simulink model "Wischer_Sensorbox"  (R2017b)
settings: Solver=FixedStepAuto  StartTime=0.0  StopTime=10.0  RelTol=1e-3
PreLoadFcn:
  | waijung.modelPreload; % Required for working with Waijung Blockset. Do not remove.
undefined symbols (not defined in the file): Blocking, HSEOSC, Link, LQFP100, Non, Raw, ST, STM32F407VG
libraries: simulink x14, hdlsllib x12, stm32f4_canbus_lib x3, stm32f4_io_lib x2, stm32f4_adc_lib x1, stm32f4_device_config_lib x1
CloseFcn:
  | waijung.modelClose; % Required for working with Waijung Blockset. Do not remove.
settings Model: Creator=Alexander  LastModifiedBy=labuser
settings OptimizationCC: DefaultParameterBehavior=Inlined
settings DebuggingCC: ParameterTunabilityLossMsg=error
settings HardwareCC: ProdBitPerPointer=32  ProdBitPerSizeT=32  ProdBitPerPtrDiffT=32  ProdLargestAtomicFloat=None  ProdIntDivRoundTo=Undefined  ProdWordSize=32  ProdHWDeviceType=ARM Compatible->Cortex - M4  TargetEndianess=LittleEndian  TargetHWDeviceType=ARM Compatible->Cortex - M4
settings SFSimCC: MATLABDynamicMemAlloc=off
settings RTWCC: SystemTargetFile=stm32f4.tlc  GenerateMakefile=off  TemplateMakefile=ert_default_tmf  Description=STM32F4 Target  GenerateReport=on  IncludeHyperlinkInReport=on  LaunchReport=on  GenerateTraceInfo=on  GenerateTraceReport=on  GenerateTraceReportSl=on  GenerateTraceReportSf=on  GenerateTraceReportEml=on
settings CodeAppCC: ForceParamTrailComments=on  IgnoreCustomStorageClasses=off  OperatorAnnotations=on  SimulinkDataObjDesc=on  SFDataObjDesc=on  MATLABFcnDesc=on  InsertBlockDesc=on  StateflowObjectComments=on  MATLABSourceComments=on
settings STFCustomTargetCC: TargetLangStandard=C99 (ISO)  ModelReferenceCompliant=off  CombineOutputUpdateFcns=on  ERTCustomFileBanners=on  SupportContinuousTime=off  SupportNonInlinedSFcns=off  RemoveResetFunc=on  MATLABClassNameForMDSCustomization=Simulink.SoftwareTarget.ERTCustomization  GRTInterface=off  SystemTargetFile=stm32f4.tlc
settings ERTTargetCC: TargetLangStandard=C99 (ISO)  MultiwordLength=2048  ModelReferenceCompliant=off  ParMdlRefBuildCompliant=off  CompOptLevelCompliant=off  ConcurrentExecutionCompliant=off  ModelStepFunctionPrototypeControlCompliant=off  CPPClassGenCompliant=off  UseToolchainInfoCompliant=off  InlinedParameterPlacement=NonHierarchical  ERTSrcFileBannerTemplate=stm32f4_code_template.cgt  ERTHdrFileBannerTemplate=stm32f4_code_template.cgt  ERTDataSrcFileTemplate=stm32f4_code_template.cgt  ERTDataHdrFileTemplate=stm32f4_code_template.cgt  ERTCustomFileTemplate=stm32f4_file_process.tlc

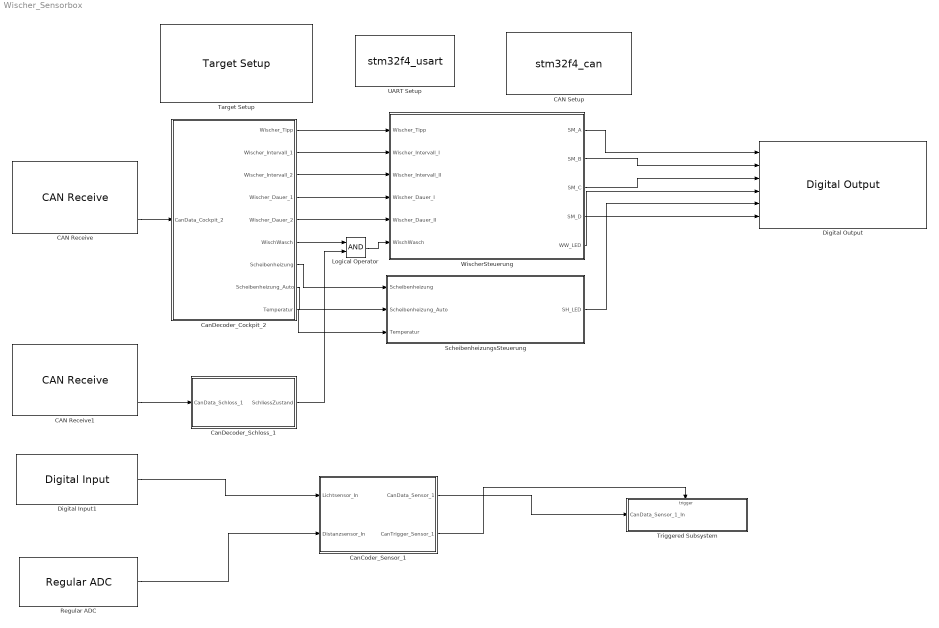
== system Wischer_Sensorbox ==
  CAN Receive : stm32f4_canbus_lib/CAN Receive  conf=Rx  canmodule=1  idtype=Standard  filtertype=Specific  id=17  idmask=0  enableisr=off  usedlc=off  datatype=single  data0type=uint16  data1type=Not used  data2type=Not used  data3type=Not used  data4type=Not used  data5type=Not used  data6type=Not used  data7type=Not used  buffersize=8  sampletime=-1  sampletimestr=-1  blockid=CANReceive  inputarray=[]  inputlabelarray={}  outputarray=[ 5, 7, 5]  outputlabelarray={ 'Msg Pending','ID', 'D0 (uint16)' }  compat=0  confstr="[\"Standard\",\"Specific\",\"17\",\"0\",\"off\",\"uint16\",\"Not used\",\"Not used\",\"Not used\",\"Not used\",\"Not used\",\"Not used\",\"Not used\",\"8\",\"220\",\"0\",\"FFE0\",\"4\"]"
  CAN Receive1 : stm32f4_canbus_lib/CAN Receive  conf=Rx  canmodule=1  idtype=Standard  filtertype=Specific  id=25  idmask=0  enableisr=off  usedlc=off  datatype=single  data0type=uint8  data1type=Not used  data2type=Not used  data3type=Not used  data4type=Not used  data5type=Not used  data6type=Not used  data7type=Not used  buffersize=8  sampletime=-1  sampletimestr=-1  blockid=CANReceive1  inputarray=[]  inputlabelarray={}  outputarray=[ 5, 7, 3]  outputlabelarray={ 'Msg Pending','ID', 'D0 (uint8)' }  compat=0  confstr="[\"Standard\",\"Specific\",\"25\",\"0\",\"off\",\"uint8\",\"Not used\",\"Not used\",\"Not used\",\"Not used\",\"Not used\",\"Not used\",\"Not used\",\"8\",\"320\",\"0\",\"FFE0\",\"4\"]"
  CAN Setup : S-Function  FunctionName=stm32f4_can  Parameters=conf,canmodule,0,inputarray,outputarray,'','',confstr,sampletime,sampletimestr,blockid  SFunctionDeploymentMode=off  EnableBusSupport=off  mask(stm32f4_can){conf=Setup, canmodule=1, advance=off, bitrate_select=125000, sjw=1tq, bs1=14tq, bs2=6tq, timingconf=Prescaler, brp=16, bitrate=125000, tq=3.8095e-07, autoretransmission=Disable, remaptxpin=D1, remaprxpin=D0, sampletime=-1, sampletimestr=-1, blockid=CANSetup, inputarray=[], inputlabelarray={}, outputarray=[], outputlabelarray={}, compat=0, confstr=["125000","16","D","1","D","0","1tq","14tq","6tq","ENABLE"], presc=16, txportstr=D, txpinstr=1, rxportstr=D, rxpinstr=0, lastmodule=1}
      mask prompts: conf "Configuration"; canmodule "CAN Module"; advance "Advance configuration"; bitrate_select "Baud rate (bps)"; sjw "Resync Jump Width (SJW)"; bs1 "Bit segment 1 (BS1) + PROP_SEG"; bs2 "Bit segment 2 (BS2)"; timingconf "Adjust"; brp "Baud rate prescaler (BRP)"; bitrate "Baud rate (bps)"; tq "Time Quantum (Second), tq"; autoretransmission "Auto Re-transmission"; remaptxpin "CAN Tx pin"; remaprxpin "CAN Rx pin"; sampletime "Sample time (sec)"; sampletimestr "Compiled sample time (sec) in string"; inputarray "Input port"; inputlabelarray "Input port label"; outputarray "Output port"; outputlabelarray "Output port label"; compat "Compatibility (Reserved for future use)"; confstr "Configuration String"; presc "Prescale"; txportstr "Tx port string"; txpinstr "Tx pin string"; rxportstr "Rx port string"; rxpinstr "Rx pin string"; lastmodule "Last module selected"
      mask help:
      | This block setups CAN Module.
      |
      | Auto Re-transmission,
      |  - Enable: The CAN hardware will automatically retransmit the message until it has been
      | successfully transmitted according to the CAN standard.
      |  - Disable: A message will be transmitted only once, independently of the transmission result
      | (successful, error or arbitration lost).
      mask init:
      | stm32f4_can_callback('init');
      mask Help: web(fullfile(waijungdocroot,'stm32f4_can_setup.htm'), '-browser')
      mask TypeOptions conf: Setup
      mask TypeOptions canmodule: 1 | 2
      mask Callback canmodule: stm32f4_can_callback('canmodule');
      mask Callback advance: stm32f4_can_callback('advance');
      mask TypeOptions bitrate_select: 125000 | 250000 | 500000 | 1000000
      mask Callback bitrate_select: stm32f4_can_callback('bitrate_select');
      mask TypeOptions sjw: 1tq | 2tq | 3tq | 4tq
      mask TypeOptions bs1: 1tq | 2tq | 3tq | 4tq | 5tq | 6tq | 7tq | 8tq | 9tq | 10tq | 11tq | 12tq | 13tq | 14tq | 15tq | 16tq
      mask Callback bs1: stm32f4_can_callback('timingconf');
      mask TypeOptions bs2: 1tq | 2tq | 3tq | 4tq | 5tq | 6tq | 7tq | 8tq
      mask Callback bs2: stm32f4_can_callback('timingconf');
      mask TypeOptions timingconf: Prescaler | Baudrate
      mask Callback timingconf: stm32f4_can_callback('timingconf');
      mask Callback brp: stm32f4_can_callback('timingconf');
      mask Callback bitrate: stm32f4_can_callback('timingconf');
      mask TypeOptions autoretransmission: Enable | Disable
      mask TypeOptions remaptxpin: Not used | A12 | B9 | D1
      mask Callback remaptxpin: stm32f4_can_callback('remaptxpin');
      mask TypeOptions remaprxpin: Not used | A11 | B8 | D0
      mask Callback remaprxpin: stm32f4_can_callback('remaprxpin');
      mask Callback sampletime: stm32f4_can_callback('sampletime');
      mask Callback sampletimestr: stm32f4_can_callback('sampletimestr');
      mask Callback blockid: stm32f4_can_callback('blockid');
      mask Display: text(0.5, 0.5, 'CAN1_Setup\nSpeed (bps): 125000\nTx/Rx pin: D1/D0','ver','middle','hor','center');
  CanCoder_Sensor_1 : Subsystem
  CanDecoder_Cockpit_2 : Subsystem
  CanDecoder_Schloss_1 : Subsystem
  Digital Input1 : stm32f4_io_lib/Digital Input  port=C  speed=100  porttype=None  porttypestr=NOPULL  use_pin0=off  use_pin1=off  use_pin2=off  use_pin3=off  use_pin4=off  use_pin5=off  use_pin6=on  use_pin7=off  use_pin8=off  use_pin9=off  use_pin10=off  use_pin11=off  use_pin12=off  use_pin13=off  use_pin14=off  use_pin15=off  pinstr=GPIO_Pin_6  usedpinarray="[0  0  0  0  0  0  1  0  0  0  0  0  0  0  0  0]"  bitbandingstr="#define DigitalInput1_C6 Peripheral_BB(GPIOC->IDR, 6)  /* Output pin */"  sampletime=0.01  sampletimestr=-1  blockid=DigitalInput1  enablecustomportlabel=off  glabalinit=off  cinputportlabel=In1, In2  coutputportlabel=Out1, Out2
  Digital Output : stm32f4_io_lib/Digital Output  use_bitband=on  port=C  speed=100  porttype=Push Pull  porttypestr=PP  use_pin0=on  use_pin1=on  use_pin2=on  use_pin3=on  use_pin4=on  use_pin5=on  use_pin6=off  use_pin7=off  use_pin8=off  use_pin9=off  use_pin10=off  use_pin11=off  use_pin12=off  use_pin13=off  use_pin14=off  use_pin15=off  pinstr=GPIO_Pin_0 | GPIO_Pin_1 | GPIO_Pin_2 | GPIO_Pin_3 | GPIO_Pin_4 | GPIO_Pin_5  usedpinarray="[1  1  1  1  1  1  0  0  0  0  0  0  0  0  0  0]"  bitbandingstr=|  sampletime=0.01  sampletimestr=-1  blockid=DigitalOutput  enablecustomportlabel=off  globalinit=off  cinputportlabel=In1, In2  coutputportlabel=0
      | #define DigitalOutput_C0 Peripheral_BB(GPIOC->ODR, 0)  /* Output pin */
      | #define DigitalOutput_C1 Peripheral_BB(GPIOC->ODR, 1)  /* Output pin */
      | #define DigitalOutput_C2 Peripheral_BB(GPIOC->ODR, 2)  /* Output pin */
      | #define DigitalOutput_C3 Peripheral_BB(GPIOC->ODR, 3)  /* Output pin */
      | #define DigitalOutput_C4 Peripheral_BB(GPIOC->ODR, 4)  /* Output pin */
      | #define DigitalOutput_C5 Peripheral_BB(GPIOC->ODR, 5)  /* Output pin */
  Logical Operator : Logic  AllPortsSameDT=off  OutDataTypeStr=boolean
  Regular ADC : stm32f4_adc_lib/Regular ADC  adcmodule=1  outputdatatype=Raw (uint16)  prescaler=2  prescalerstr=ADC_Prescaler_Div2  chsamplingtime=Auto  chsamplingtimestr=ADC_SampleTime_480Cycles  read_an0=on  read_an1=off  read_an2=off  read_an3=off  read_an4=off  read_an5=off  read_an6=off  read_an7=off  read_an8=off  read_an9=off  read_an10=off  read_an11=off  read_an12=off  read_an13=off  read_an14=off  read_an15=off  read_an16=off  read_an17=off  read_an18=off  pinstr=GPIO_Pin_0  usedpinarray="[1  0  0  0  0  0  0  0  0  0  0  0  0  0  0  0  0  0  0]"  usedportidarray=[0]  usedpinidarray=[0]  usedpinidcount=1  sampletime=0.01  blockid=RegularADC  enablecustomportlabel=off  cinputportlabel=0  coutputportlabel=Out1, Out2
  ScheibenheizungsSteuerung : Stateflow chart  TreatAsAtomicUnit=on
  Target Setup : stm32f4_device_config_lib/Target Setup  Priority=100  compiler=GNU ARM  previous_compiler=GNU ARM  mcu=STM32F407VG (LQFP100)  mcustr=STM32F407VG  clockconfig=HSEOSC-8MHz  system_stm32f4xx_c_path=C:\Users\labuser\Desktop\waijung17_03a\targets\stm32f4_target\stm32f4\utils\system_stm32f4xx_default\STM32F40_41xxx\hseosc8mhz  showmemoryconfiguration=off  stacksize=0x2000  heapsize=0x2000  enableautocompiledownload=on  fullchiperase=off  programmerinterface=ST-Link  editctrlstr=on  compilercontrolstr=$(patsubst %, -I%, .) -mcpu=cortex-m4 -mthumb -mthumb-interwork -mfloat-abi=hard -mfpu=fpv4-sp-d16 -ffast-math -Wall -Wextra -Ofast  assemblercontrolstr=$(patsubst %, -I%, .) -mcpu=cortex-m4 -mthumb -mthumb-interwork -mfloat-abi=hard -mfpu=fpv4-sp-d16 -ffast-math -Wall -Wextra -Ofast -Wa,-amhls=$(<:.s=.lst) -D__STACK_SIZE=$(STACK_SIZE) -D__HEAP_SIZE=$(HEAP_SIZE)  linkercontrolstr=-T$(LD_SCRIPT) -g -Wl,-Map=$(MAP),--cref,--no-warn-mismatch -mcpu=cortex-m4 -mthumb -mthumb-interwork -mfloat-abi=hard -mfpu=fpv4-sp-d16 -specs=nosys.specs  runafterdownload=on  execprofile=None  profileruart=3  profilerbaud=500000  profilertxpin=D8  profilerinitstr=0.01,168000000,1680000,500000,0  manualsetsampletime=off  sampletime=0.01  blockid=TargetSetup  systickreloadvalue=1680000  hseval=8000000  lastprofileruart=3  hclk=168000000  flashorigin=0x8000000  flashlength=1024k  ramorigin=0x20000000  ramlength=128k  useextram=off
  Triggered Subsystem : Subsystem  TreatAsAtomicUnit=on
  UART Setup : S-Function  Priority=1  FunctionName=stm32f4_usart  Parameters=configuration,uartmodule,transfer,baudrate,inputtype,outputtype,confstr,binheaderarray,binterminatorarray,asciiheader,asciiterminator,bindatalength,packetmode,varname,sampletime,sampletimestr,blockid  SFunctionDeploymentMode=off  EnableBusSupport=off  mask(stm32f4_usart){configuration=Setup, uartmodule=2, baudrate=115200, databits=8, parity=No, stopbit=1, remaptxpin=A2, remaprxpin=A3, flowcontrol=None, remapctspin=Not used, remaprtspin=Not used, advanceoptions=off, rxbuffersize=512, txbuffersize=512, transfer=Blocking, packetmode=Ascii, binheader='7E 7E', binterminator='03 03', porttype_double=1, porttype_single=0, porttype_int8=1, porttype_uint8=0, porttype_int16=0, porttype_uint16=0, porttype_int32=0, porttype_uint32=0, asciiformat='%d,%f', rx_asciiterminator=CRLF (0x0D 0x0A - "\r\n"), tx_asciiterminator=CR (0x0D - "\r"), storagename=<empty>, varname=, inputtype=[0], outputtype=[0], binheaderarray=[0], binterminatorarray=[0], bindatalength=0, asciiheader='', asciiterminator=[0], sampletime=-1, sampletimestr=-1, blockid=UARTSetup, confstr=[ "dummy", "1", "A", "2", "1", "A", "3", "0", "*", "*", "0", "*", "*", "1", "4", "6", "1", "4", "5", "512", "512", "1", "2", "115200", "8", "No", "1", "None", "USART2"], lastmodule=2}
      mask prompts: uartmodule "UART Module"; baudrate "Baud rate (bps)"; databits "Data bits"; stopbit "Stop bit"; remaptxpin "Tx Pin"; remaprxpin "Rx Pin"; flowcontrol "Hardware flow control"; remapctspin "HW Flow control, CTS Pin"; remaprtspin "HW Flow control, RTS Pin"; advanceoptions "Advance options"; rxbuffersize "Rx buffer size (bytes)"; txbuffersize "Tx buffer size (bytes)"; packetmode "Packet mode"; binheader "Binary header (example: '7E 7E')"; binterminator "Binary terminator (example: '03 03')"; porttype_double "Number of data port, type DOUBLE"; porttype_single "Number of data port, type SINGLE"; porttype_int8 "Number of data port, type INT8"; porttype_uint8 "Number of data port, type UINT8"; porttype_int16 "Number of data port, type INT16"; porttype_uint16 "Number of data port, type UINT16"; porttype_int32 "Number of data port, type INT32"; porttype_uint32 "Number of data port, type UINT32"; asciiformat "Ascii format"; rx_asciiterminator "End of packet"; tx_asciiterminator "End of packet"; storagename "Buffer"; varname "Var name"; inputtype "Input data type"; outputtype "Output data type"; binheaderarray "Binary header"; binterminatorarray "Binary terminator"; bindatalength "Binary data length"; asciiheader "Ascii header (printf format)"; asciiterminator "Ascii terminator"; sampletime "Sample time (sec)"; sampletimestr "Compiled sample time (sec) in string"; confstr "Configuration string"; lastmodule "Last module selected"
      mask help:
      | Default STM32F4DISCOVERY + aMG F4 Connect 2 + aMG USB Converter N2 settings use
      |
      | USART3, Tx D8, Rx D9 and USB Serial Converter A.
      mask init:
      | stm32f4_usart_callback('init');
      mask Help: web(fullfile(waijungdocroot,'stm32f4_usart_setup.htm'), '-browser')
      mask TypeOptions configuration: Setup | Tx | Rx
      mask Callback configuration: stm32f4_usart_callback('configuration');
      mask TypeOptions uartmodule: 1 | 2 | 3 | 4 | 5 | 6
      mask Callback uartmodule: stm32f4_usart_callback('uartmodule');
      mask Callback baudrate: stm32f4_usart_callback('baudrate');
      mask TypeOptions databits: 8
      mask TypeOptions parity: No | Odd | Even
      mask TypeOptions stopbit: 0.5 | 1 | 1.5 | 2
      mask TypeOptions remaptxpin: Not used | A2 | D5
      mask TypeOptions remaprxpin: Not used | A3 | D6
      mask TypeOptions flowcontrol: None | RTS | CTS | RTS/CTS
      mask Callback flowcontrol: stm32f4_usart_callback('flowcontrol');
      mask TypeOptions remapctspin: Not used | A0 | D3
      mask TypeOptions remaprtspin: Not used | A1 | D4
      mask Callback advanceoptions: stm32f4_usart_callback('advanceoptions');
      mask TypeOptions rxbuffersize: 16 | 32 | 64 | 128 | 256 | 512 | 1024 | 2048
      mask TypeOptions txbuffersize: 16 | 32 | 64 | 128 | 256 | 512 | 1024 | 2048
      mask TypeOptions transfer: Blocking | Non-Blocking
      mask Callback transfer: stm32f4_usart_callback('transfer');
      mask TypeOptions packetmode: Ascii | Binary | String Buffer
      mask Callback packetmode: stm32f4_usart_callback('packetmode');
      mask Callback binheader: stm32f4_usart_callback('binheader');
      mask Callback binterminator: stm32f4_usart_callback('binterminator');
      mask Callback porttype_double: stm32f4_usart_callback('porttype');
      mask Callback porttype_single: stm32f4_usart_callback('porttype');
      mask Callback porttype_int8: stm32f4_usart_callback('porttype');
      mask Callback porttype_uint8: stm32f4_usart_callback('porttype');
      mask Callback porttype_int16: stm32f4_usart_callback('porttype');
      mask Callback porttype_uint16: stm32f4_usart_callback('porttype');
      mask Callback porttype_int32: stm32f4_usart_callback('porttype');
      mask Callback porttype_uint32: stm32f4_usart_callback('porttype');
      mask Callback asciiformat: stm32f4_usart_callback('asciiformat');
      mask TypeOptions rx_asciiterminator: CR (0x0D - "\r") | LF (0x0A - "\n") | CRLF (0x0D 0x0A - "\r\n")
      mask Callback rx_asciiterminator: stm32f4_usart_callback('rx_asciiterminator');
      mask TypeOptions tx_asciiterminator: CR (0x0D - "\r") | LF (0x0A - "\n") | CRLF (0x0D 0x0A - "\r\n") | None
      mask Callback tx_asciiterminator: stm32f4_usart_callback('tx_asciiterminator');
      mask TypeOptions storagename: <empty>
      mask Callback storagename: stm32f4_usart_callback('storagename');
      mask Callback varname: stm32f4_usart_callback('varname');
      mask Callback sampletime: stm32f4_usart_callback('sampletime');
      mask Callback sampletimestr: stm32f4_usart_callback('sampletimestr');
      mask Callback blockid: stm32f4_usart_callback('blockid');
      mask Display: text(0.5, 0.5, 'Module: USART2_Setup\nBaud (Bps): 115200\nDMA Buffer: 512/512\nTx/Rx Pin: A2/A3','ver','middle','hor','center');
  WischerSteuerung : Stateflow chart  TreatAsAtomicUnit=on
  wires:
  ScheibenheizungsSteuerung/1(SH_LED) -> Digital Output/5
  CanDecoder_Cockpit_2/9(Temperatur) -> ScheibenheizungsSteuerung/3(Temperatur)
  CanDecoder_Cockpit_2/3(Wischer_Intervall_2) -> WischerSteuerung/3(Wischer_Intervall_II)
  CanDecoder_Cockpit_2/7(Scheibenheizung) -> ScheibenheizungsSteuerung/1(Scheibenheizung)
  CanDecoder_Cockpit_2/5(Wischer_Dauer_2) -> WischerSteuerung/5(Wischer_Dauer_II)
  CanDecoder_Cockpit_2/2(Wischer_Intervall_1) -> WischerSteuerung/2(Wischer_Intervall_I)
  CanDecoder_Cockpit_2/8(Scheibenheizung_Auto) -> ScheibenheizungsSteuerung/2(Scheibenheizung_Auto)
  WischerSteuerung/5(WW_LED) -> Digital Output/6
  CanDecoder_Cockpit_2/4(Wischer_Dauer_1) -> WischerSteuerung/4(Wischer_Dauer_I)
  WischerSteuerung/4(SM_D) -> Digital Output/4
  WischerSteuerung/3(SM_C) -> Digital Output/3
  WischerSteuerung/2(SM_B) -> Digital Output/2
  WischerSteuerung/1(SM_A) -> Digital Output/1
  CanDecoder_Cockpit_2/1(Wischer_Tipp) -> WischerSteuerung/1(Wischer_Tipp)
  CAN Receive/3 -> CanDecoder_Cockpit_2/1(CanData_Cockpit_2)
  CAN Receive1/3 -> CanDecoder_Schloss_1/1(CanData_Schloss_1)
  CanDecoder_Cockpit_2/6(WischWasch) -> Logical Operator/1
  Logical Operator/1 -> WischerSteuerung/6(WischWasch)
  CanDecoder_Schloss_1/1(SchliessZustand) -> Logical Operator/2
  Digital Input1/1 -> CanCoder_Sensor_1/1(Lichtsensor_In)
  Regular ADC/1 -> CanCoder_Sensor_1/2(Distanzsensor_In)
  CanCoder_Sensor_1/1(CanData_Sensor_1) -> Triggered Subsystem/1(CanData_Sensor_1_In)
  CanCoder_Sensor_1/2(CanTrigger_Sensor_1) -> Triggered Subsystem/Trigger

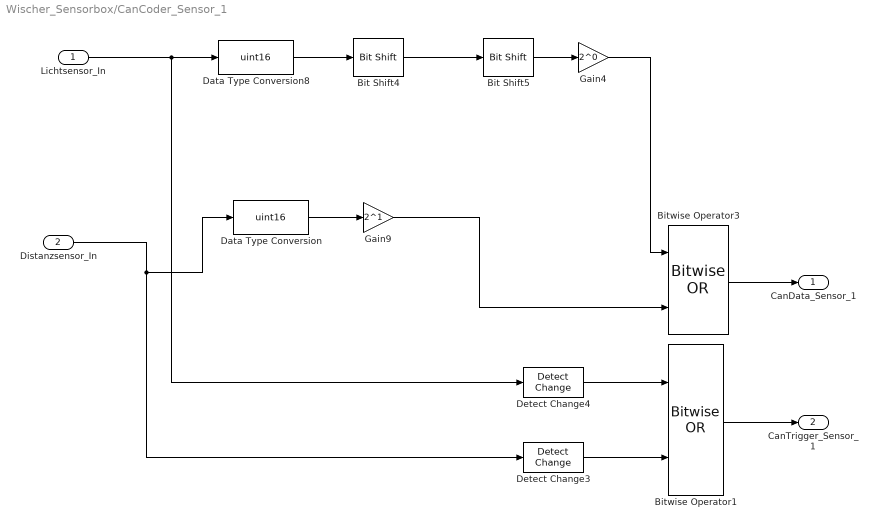
== system Wischer_Sensorbox/CanCoder_Sensor_1 ==
  Lichtsensor_In : Inport
  Distanzsensor_In : Inport  Port=2
  Bit Shift4 : hdlsllib/Logic and Bit Operations/Bit Shift  mode=Shift Left Logical  N=7
      settings: SourceProductName=HDL Coder  SourceProductBaseCode=HD
  Bit Shift5 : hdlsllib/Logic and Bit Operations/Bit Shift  mode=Shift Right Logical  N=7
      settings: SourceProductName=HDL Coder  SourceProductBaseCode=HD
  Bitwise Operator1 : simulink/Logic and Bit Operations/Bitwise Operator  logicop=OR  UseBitMask=off  NumInputPorts=2  BitMask=bin2dec('11011001')  BitMaskRealWorld=Stored Integer
  Bitwise Operator3 : simulink/Logic and Bit Operations/Bitwise Operator  logicop=OR  UseBitMask=off  NumInputPorts=2  BitMask=bin2dec('11011001')  BitMaskRealWorld=Stored Integer
  Data Type Conversion : DataTypeConversion  OutDataTypeStr=uint16
  Data Type Conversion8 : DataTypeConversion  OutDataTypeStr=uint16
  Detect Change3 : simulink/Logic and Bit Operations/Detect Change  vinit=0  OutDataTypeStr=boolean
  Detect Change4 : simulink/Logic and Bit Operations/Detect Change  vinit=0  OutDataTypeStr=boolean
  Gain4 : Gain  Gain=2^0  OutDataTypeStr=uint16
  Gain9 : Gain  Gain=2^1  OutDataTypeStr=uint16
  CanData_Sensor_1 : Outport
  CanTrigger_Sensor_1 : Outport  Port=2
  wires:
  Bitwise Operator1/1 -> CanTrigger_Sensor_1/1
  Bitwise Operator3/1 -> CanData_Sensor_1/1
  Data Type Conversion/1 -> Gain9/1
  Gain4/1 -> Bitwise Operator3/1
  Detect Change3/1 -> Bitwise Operator1/2
  Lichtsensor_In/1 -> Data Type Conversion8/1, Detect Change4/1
  Distanzsensor_In/1 -> Data Type Conversion/1, Detect Change3/1
  Gain9/1 -> Bitwise Operator3/2
  Detect Change4/1 -> Bitwise Operator1/1
  Bit Shift4/1 -> Bit Shift5/1
  Data Type Conversion8/1 -> Bit Shift4/1
  Bit Shift5/1 -> Gain4/1

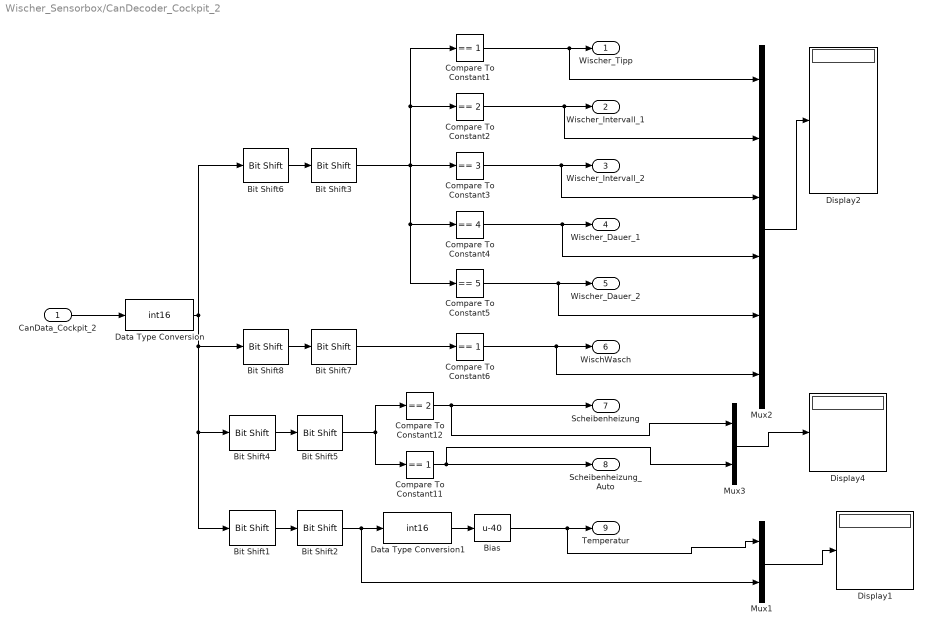
== system Wischer_Sensorbox/CanDecoder_Cockpit_2 ==
  CanData_Cockpit_2 : Inport
  Bias : Bias  Bias=-40
  Bit Shift1 : hdlsllib/Logic and Bit Operations/Bit Shift  mode=Shift Left Logical  N=3
      settings: SourceProductName=HDL Coder  SourceProductBaseCode=HD
  Bit Shift2 : hdlsllib/Logic and Bit Operations/Bit Shift  mode=Shift Right Logical  N=9
      settings: SourceProductName=HDL Coder  SourceProductBaseCode=HD
  Bit Shift3 : hdlsllib/Logic and Bit Operations/Bit Shift  mode=Shift Right Logical  N=13
      settings: SourceProductName=HDL Coder  SourceProductBaseCode=HD
  Bit Shift4 : hdlsllib/Logic and Bit Operations/Bit Shift  mode=Shift Left Logical  N=10
      settings: SourceProductName=HDL Coder  SourceProductBaseCode=HD
  Bit Shift5 : hdlsllib/Logic and Bit Operations/Bit Shift  mode=Shift Right Logical  N=14
      settings: SourceProductName=HDL Coder  SourceProductBaseCode=HD
  Bit Shift6 : hdlsllib/Logic and Bit Operations/Bit Shift  mode=Shift Left Logical  N=13
      settings: SourceProductName=HDL Coder  SourceProductBaseCode=HD
  Bit Shift7 : hdlsllib/Logic and Bit Operations/Bit Shift  mode=Shift Right Logical  N=15
      settings: SourceProductName=HDL Coder  SourceProductBaseCode=HD
  Bit Shift8 : hdlsllib/Logic and Bit Operations/Bit Shift  mode=Shift Left Logical  N=12
      settings: SourceProductName=HDL Coder  SourceProductBaseCode=HD
  Compare To Constant1 : simulink/Logic and Bit Operations/Compare To Constant  relop===  const=1  OutDataTypeStr=uint8
  Compare To Constant11 : simulink/Logic and Bit Operations/Compare To Constant  relop===  const=1  OutDataTypeStr=uint8
  Compare To Constant12 : simulink/Logic and Bit Operations/Compare To Constant  relop===  const=2  OutDataTypeStr=uint8
  Compare To Constant2 : simulink/Logic and Bit Operations/Compare To Constant  relop===  const=2  OutDataTypeStr=uint8
  Compare To Constant3 : simulink/Logic and Bit Operations/Compare To Constant  relop===  const=3  OutDataTypeStr=uint8
  Compare To Constant4 : simulink/Logic and Bit Operations/Compare To Constant  relop===  const=4  OutDataTypeStr=uint8
  Compare To Constant5 : simulink/Logic and Bit Operations/Compare To Constant  relop===  const=5  OutDataTypeStr=uint8
  Compare To Constant6 : simulink/Logic and Bit Operations/Compare To Constant  relop===  const=1  OutDataTypeStr=uint8
  Data Type Conversion : DataTypeConversion  OutDataTypeStr=int16
  Data Type Conversion1 : DataTypeConversion  OutDataTypeStr=int16
  Display1 : Display
  Display2 : Display
  Display4 : Display
  Mux1 : Mux  Inputs=2
  Mux2 : Mux  Inputs=6
  Mux3 : Mux  Inputs=2
  Wischer_Tipp : Outport
  Wischer_Intervall_1 : Outport  Port=2
  Wischer_Intervall_2 : Outport  Port=3
  Wischer_Dauer_1 : Outport  Port=4
  Wischer_Dauer_2 : Outport  Port=5
  WischWasch : Outport  Port=6
  Scheibenheizung : Outport  Port=7
  Scheibenheizung_Auto : Outport  Port=8
  Temperatur : Outport  Port=9
  wires:
  Mux3/1 -> Display4/1
  Bit Shift5/1 -> Compare To Constant11/1, Compare To Constant12/1
  Bit Shift4/1 -> Bit Shift5/1
  Compare To Constant11/1 -> Mux3/2, Scheibenheizung_Auto/1
  CanData_Cockpit_2/1 -> Data Type Conversion/1
  Compare To Constant12/1 -> Mux3/1, Scheibenheizung/1
  Bit Shift1/1 -> Bit Shift2/1
  Data Type Conversion/1 -> Bit Shift1/1, Bit Shift4/1, Bit Shift8/1, Bit Shift6/1
  Bit Shift2/1 -> Mux1/2, Data Type Conversion1/1
  Bias/1 -> Mux1/1, Temperatur/1
  Data Type Conversion1/1 -> Bias/1
  Mux1/1 -> Display1/1
  Bit Shift6/1 -> Bit Shift3/1
  Mux2/1 -> Display2/1
  Bit Shift3/1 -> Compare To Constant5/1, Compare To Constant4/1, Compare To Constant3/1, Compare To Constant2/1, Compare To Constant1/1
  Compare To Constant1/1 -> Mux2/1, Wischer_Tipp/1
  Compare To Constant2/1 -> Mux2/2, Wischer_Intervall_1/1
  Compare To Constant3/1 -> Mux2/3, Wischer_Intervall_2/1
  Compare To Constant4/1 -> Mux2/4, Wischer_Dauer_1/1
  Compare To Constant5/1 -> Mux2/5, Wischer_Dauer_2/1
  Compare To Constant6/1 -> Mux2/6, WischWasch/1
  Bit Shift8/1 -> Bit Shift7/1
  Bit Shift7/1 -> Compare To Constant6/1

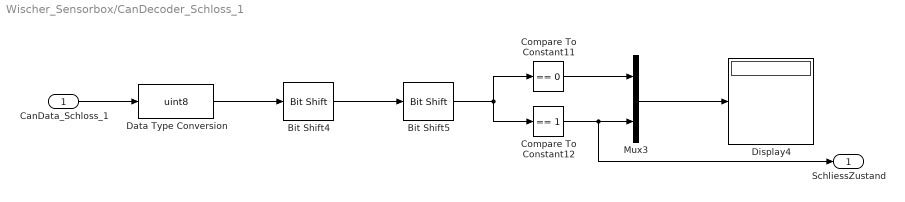
== system Wischer_Sensorbox/CanDecoder_Schloss_1 ==
  CanData_Schloss_1 : Inport
  Bit Shift4 : hdlsllib/Logic and Bit Operations/Bit Shift  mode=Shift Left Logical  N=7
      settings: SourceProductName=HDL Coder  SourceProductBaseCode=HD
  Bit Shift5 : hdlsllib/Logic and Bit Operations/Bit Shift  mode=Shift Right Logical  N=7
      settings: SourceProductName=HDL Coder  SourceProductBaseCode=HD
  Compare To Constant11 : simulink/Logic and Bit Operations/Compare To Constant  relop===  const=0  OutDataTypeStr=boolean
  Compare To Constant12 : simulink/Logic and Bit Operations/Compare To Constant  relop===  const=1  OutDataTypeStr=boolean
  Data Type Conversion : DataTypeConversion  OutDataTypeStr=uint8
  Display4 : Display
  Mux3 : Mux  Inputs=2
  SchliessZustand : Outport
  wires:
  Mux3/1 -> Display4/1
  Compare To Constant11/1 -> Mux3/1
  Compare To Constant12/1 -> SchliessZustand/1, Mux3/2
  Bit Shift4/1 -> Bit Shift5/1
  Bit Shift5/1 -> Compare To Constant11/1, Compare To Constant12/1
  Data Type Conversion/1 -> Bit Shift4/1
  CanData_Schloss_1/1 -> Data Type Conversion/1

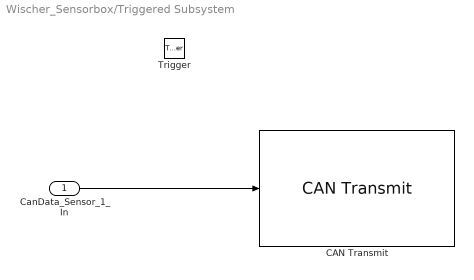
== system Wischer_Sensorbox/Triggered Subsystem ==
  CanData_Sensor_1_In : Inport
  Trigger : TriggerPort  VariantControl=Variant
  CAN Transmit : stm32f4_canbus_lib/CAN Transmit  conf=Tx  canmodule=1  transfer=Non-Blocking  timeout=0.005  idtype=Standard  specificid=on  id=32  specificdlc=on  dlc=2  enablestatus=off  datatype=single  data0type=uint16  data1type=Not used  data2type=Not used  data3type=Not used  data4type=Not used  data5type=Not used  data6type=Not used  data7type=Not used  inputarray=[ 5]  inputlabelarray={ 'D0 (uint16)' }  outputarray=[]  outputlabelarray={}  sampletime=-1  sampletimestr=-1  blockid=TriggeredSubsystemCANTransmit  compat=0  confstr="[\"Non-Blocking\",\"0.005\",\"Standard\",\"on\",\"32\",\"on\",\"2\",\"off\",\"uint16\",\"Not used\",\"Not used\",\"Not used\",\"Not used\",\"Not used\",\"Not used\",\"Not used\"]"
  wires:
  CanData_Sensor_1_In/1 -> CAN Transmit/1

== stateflow chart Wischer_Sensorbox/WischerSteuerung ==
  state Wischer [commented out]
    state Stufe_0_ [commented out]
      entry:
      SM_A=false
      SM_B=false
      SM_C=false
      SM_D=false
      WW_LED=false
      Steps=0
      WischWaschCount=0
    state Wischer_Vor [commented out]
      state Phase4 [commented out]
        entry:
        SM_A=false
        SM_B=false
        SM_C=false
        SM_D=true
        WW_LED=false
        Steps = Steps + 1;
      state Phase1 [commented out]
        entry:
        SM_A=true
        SM_B=false
        SM_C=false
        SM_D=false
        WW_LED=false
        Steps = Steps + 1;
      state Phase2 [commented out]
        entry:
        SM_A=false
        SM_B=true
        SM_C=false
        SM_D=false
        WW_LED=false
        Steps = Steps+1;
      state Phase3 [commented out]
        entry:
        SM_A=false
        SM_B=false
        SM_C=true
        SM_D=false
        WW_LED=false
        Steps = Steps+1;
      (default) -> Wischer.Wischer_Vor.Phase1 [commented out]
      Wischer.Wischer_Vor.Phase4 -> Wischer.Wischer_Vor.Phase1 [commented out] : after(StepTime,sec)
      Wischer.Wischer_Vor.Phase1 -> Wischer.Wischer_Vor.Phase2 [commented out] : after(StepTime,sec)
      Wischer.Wischer_Vor.Phase3 -> Wischer.Wischer_Vor.Phase4 [commented out] : after(StepTime,sec)
      Wischer.Wischer_Vor.Phase2 -> Wischer.Wischer_Vor.Phase3 [commented out] : after(StepTime,sec)
    state TIPP [commented out]
      entry: StepTime=0.0303;
      StepTime1=1;
      BreakTime=1;
    state INTERVALL_LANGSAM [commented out]
      entry: StepTime=0.0303;
      StepTime1=1;
      BreakTime=4;
    state INTERVALL_LANGSAM1 [commented out]
      entry: StepTime=0.0303;
      StepTime1=1;
      BreakTime=2;
    state Warte [commented out]
    state Wischer_Rueck [commented out]
      state Phase4 [commented out]
        entry:
        SM_A=false
        SM_B=false
        SM_C=false
        SM_D=true
        WW_LED=false
        Steps = Steps+1;
      state Phase1 [commented out]
        entry:
        SM_A=true
        SM_B=false
        SM_C=false
        SM_D=false
        WW_LED=false
        Steps = Steps+1;
      state Phase2 [commented out]
        entry:
        SM_A=false
        SM_B=true
        SM_C=false
        SM_D=false
        WW_LED=false
        Steps = Steps+1;
      state Phase3 [commented out]
        entry:
        SM_A=false
        SM_B=false
        SM_C=true
        SM_D=false
        WW_LED=false
        Steps = Steps+1;
      Wischer.Wischer_Rueck.Phase1 -> Wischer.Wischer_Rueck.Phase4 [commented out] : after(StepTime,sec)
      (default) -> Wischer.Wischer_Rueck.Phase4 [commented out]
      Wischer.Wischer_Rueck.Phase2 -> Wischer.Wischer_Rueck.Phase1 [commented out] : after(StepTime,sec)
      Wischer.Wischer_Rueck.Phase4 -> Wischer.Wischer_Rueck.Phase3 [commented out] : after(StepTime,sec)
      Wischer.Wischer_Rueck.Phase3 -> Wischer.Wischer_Rueck.Phase2 [commented out] : after(StepTime,sec)
    (default) -> Wischer.Stufe_0_ [commented out]
    Wischer.Stufe_0_ -> Wischer.TIPP [commented out] : [Wischer_Tipp==1]
    Wischer.TIPP -> Wischer.Wischer_Vor [commented out]
    Wischer.Stufe_0_ -> Wischer.INTERVALL_LANGSAM [commented out] : [Wischer_Intervall_I==1]
    Wischer.INTERVALL_LANGSAM -> Wischer.Wischer_Vor [commented out]
    Wischer.Stufe_0_ -> Wischer.INTERVALL_LANGSAM1 [commented out] : [Wischer_Intervall_II==1]
    Wischer.INTERVALL_LANGSAM1 -> Wischer.Wischer_Vor [commented out]
    Wischer.Wischer_Rueck -> Warte [commented out] : [Steps==66]
    Warte -> Wischer.Stufe_0_ [commented out] : after(BreakTime,sec)
    Wischer.Wischer_Vor -> Wischer.Wischer_Rueck [commented out] : [Steps==33]
  state Wischer1
    state Stufe_0_
      entry:
      SM_A=false
      SM_B=false
      SM_C=false
      SM_D=false
      WW_LED=false
      Steps=0
      WischWaschCount=0
    state Wischer_Vor
      state Phase4
        entry:
        SM_A=false
        SM_B=false
        SM_C=false
        SM_D=true
        WW_LED=false
        Steps = Steps + 1;
      state Phase1
        entry:
        SM_A=true
        SM_B=false
        SM_C=false
        SM_D=false
        WW_LED=false
        Steps = Steps + 1;
      state Phase2
        entry:
        SM_A=false
        SM_B=true
        SM_C=false
        SM_D=false
        WW_LED=false
        Steps = Steps + 1;
      state Phase3
        entry:
        SM_A=false
        SM_B=false
        SM_C=true
        SM_D=false
        WW_LED=false
        Steps = Steps + 1;
      (default) -> Wischer1.Wischer_Vor.Phase1
      Wischer1.Wischer_Vor.Phase4 -> Wischer1.Wischer_Vor.Phase1 : after(StepTime,sec)
      Wischer1.Wischer_Vor.Phase1 -> Wischer1.Wischer_Vor.Phase2 : after(StepTime,sec)
      Wischer1.Wischer_Vor.Phase3 -> Wischer1.Wischer_Vor.Phase4 : after(StepTime,sec)
      Wischer1.Wischer_Vor.Phase2 -> Wischer1.Wischer_Vor.Phase3 : after(StepTime,sec)
    state TIPP
      entry: StepTime=0.0303;
      StepTime1=1;
      BreakTime=1;
    state INTERVALL_LANGSAM
      entry: StepTime=0.0303;
      StepTime1=1;
      BreakTime=4;
    state INTERVALL_LANGSAM1
      entry: StepTime=0.0303;
      StepTime1=1;
      BreakTime=2;
    state INTERVALL_LANGSAM2
      entry: StepTime=0.0303;
      StepTime1=1;
      BreakTime=0;
    state INTERVALL_LANGSAM3
      entry: StepTime=0.015015;
      StepTime1=0.5;
      BreakTime=0;
    state WEIL_ICH_DUMM_BIN
    state Wischer_Rueck
      state Phase4
        entry:
        SM_A=false
        SM_B=false
        SM_C=false
        SM_D=true
        WW_LED=false
        Steps = Steps - 1;
      state Phase1
        entry:
        SM_A=true
        SM_B=false
        SM_C=false
        SM_D=false
        WW_LED=false
        Steps = Steps -1;
      state Phase2
        entry:
        SM_A=false
        SM_B=true
        SM_C=false
        SM_D=false
        WW_LED=false
        Steps = Steps - 1;
      state Phase3
        entry:
        SM_A=false
        SM_B=false
        SM_C=true
        SM_D=false
        WW_LED=false
        Steps = Steps - 1;
      (default) -> Wischer1.Wischer_Rueck.Phase4
      Wischer1.Wischer_Rueck.Phase1 -> Wischer1.Wischer_Rueck.Phase4 : after(StepTime,sec)
      Wischer1.Wischer_Rueck.Phase2 -> Wischer1.Wischer_Rueck.Phase1 : after(StepTime,sec)
      Wischer1.Wischer_Rueck.Phase4 -> Wischer1.Wischer_Rueck.Phase3 : after(StepTime,sec)
      Wischer1.Wischer_Rueck.Phase3 -> Wischer1.Wischer_Rueck.Phase2 : after(StepTime,sec)
    (default) -> Wischer1.Stufe_0_
    Wischer1.Stufe_0_ -> Wischer1.TIPP [order 1] : [Wischer_Tipp==1]
    Wischer1.TIPP -> Wischer1.Wischer_Vor
    Wischer1.Stufe_0_ -> Wischer1.INTERVALL_LANGSAM [order 2] : [Wischer_Intervall_I==1]
    Wischer1.INTERVALL_LANGSAM -> Wischer1.Wischer_Vor
    Wischer1.Stufe_0_ -> Wischer1.INTERVALL_LANGSAM1 [order 5] : [Wischer_Intervall_II==1]
    Wischer1.INTERVALL_LANGSAM1 -> Wischer1.Wischer_Vor
    INTERVALL_LANGSAM2 -> Wischer1.Wischer_Vor
    Wischer1.Stufe_0_ -> INTERVALL_LANGSAM2 [order 3] : [Wischer_Dauer_I==1]
    Wischer1.Stufe_0_ -> INTERVALL_LANGSAM3 [order 4] : [Wischer_Dauer_II==1]
    INTERVALL_LANGSAM3 -> Wischer1.Wischer_Vor
    WEIL_ICH_DUMM_BIN -> Wischer1.Stufe_0_ : after(BreakTime,sec)
    Wischer1.Wischer_Rueck -> WEIL_ICH_DUMM_BIN : [Steps==0]
    Wischer1.Wischer_Vor -> Wischer1.Wischer_Rueck : [Steps==23]
  state WischWasch [group]
    state Wischer_Vor_WW
      state Phase4
        entry:
        SM_A=false
        SM_B=false
        SM_C=false
        SM_D=true
        WW_LED=false
        Steps = Steps + 1;
      state Phase1
        entry:
        SM_A=true
        SM_B=false
        SM_C=false
        SM_D=false
        WW_LED=false
        Steps = Steps + 1;
      state Phase2
        entry:
        SM_A=false
        SM_B=true
        SM_C=false
        SM_D=false
        WW_LED=false
        Steps = Steps + 1;
      state Phase3
        entry:
        SM_A=false
        SM_B=false
        SM_C=true
        SM_D=false
        WW_LED=false
        Steps = Steps + 1;
      (default) -> WischWasch.Wischer_Vor_WW.Phase1
      WischWasch.Wischer_Vor_WW.Phase4 -> WischWasch.Wischer_Vor_WW.Phase1 : after(StepTime,sec)
      WischWasch.Wischer_Vor_WW.Phase1 -> WischWasch.Wischer_Vor_WW.Phase2 : after(StepTime,sec)
      WischWasch.Wischer_Vor_WW.Phase3 -> WischWasch.Wischer_Vor_WW.Phase4 : after(StepTime,sec)
      WischWasch.Wischer_Vor_WW.Phase2 -> WischWasch.Wischer_Vor_WW.Phase3 : after(StepTime,sec)
    state Spruehen
      entry:WW_LED=true
      WischWaschCount=2
      StepTime=1/33
      exit: WW_LED=false
    state Wischer_Rueck_WW
      state Phase4
        entry:
        SM_A=false
        SM_B=false
        SM_C=false
        SM_D=true
        WW_LED=false
        Steps = Steps - 1;
      state Phase1
        entry:
        SM_A=true
        SM_B=false
        SM_C=false
        SM_D=false
        WW_LED=false
        Steps = Steps -1;
      state Phase2
        entry:
        SM_A=false
        SM_B=true
        SM_C=false
        SM_D=false
        WW_LED=false
        Steps = Steps - 1;
      state Phase3
        entry:
        SM_A=false
        SM_B=false
        SM_C=true
        SM_D=false
        WW_LED=false
        Steps = Steps - 1;
      (default) -> WischWasch.Wischer_Rueck_WW.Phase1
      WischWasch.Wischer_Rueck_WW.Phase1 -> WischWasch.Wischer_Rueck_WW.Phase4 : after(StepTime,sec)
      WischWasch.Wischer_Rueck_WW.Phase2 -> WischWasch.Wischer_Rueck_WW.Phase1 : after(StepTime,sec)
      WischWasch.Wischer_Rueck_WW.Phase4 -> WischWasch.Wischer_Rueck_WW.Phase3 : after(StepTime,sec)
      WischWasch.Wischer_Rueck_WW.Phase3 -> WischWasch.Wischer_Rueck_WW.Phase2 : after(StepTime,sec)
    Wischer_Rueck_WW -> Wischer_Vor_WW [order 1] : [Steps==0&&WischWaschCount>0 ]{WischWaschCount = WischWaschCount - 1}
    Spruehen -> Wischer_Vor_WW : after(2,sec)
    Wischer_Vor_WW -> Wischer_Rueck_WW : [Steps==23]
  (default) -> Wischer [commented out]
  (default) -> Wischer1
  Wischer1 -> Spruehen : [WischWasch==1 &&Steps==0]
  Wischer_Rueck_WW -> Wischer1 [order 2] : [WischWaschCount==0&&Steps==0]
  data: Wischer_Tipp input; Wischer_Intervall_I input; Wischer_Intervall_II input; Wischer_Dauer_I input; Wischer_Dauer_II input; WischWasch input; SM_A output; SM_B output; SM_C output; SM_D output; WW_LED output; Steps local; Forward local; StepTime local; StepTime1 local; Count local double; BreakTime local; Rueck local boolean; WischWaschCount local uint8

== stateflow chart Wischer_Sensorbox/ScheibenheizungsSteuerung ==
  state MANUELL
    state ON
      entry:SH_LED=true
    state OFF
      entry:SH_LED=false
    (default) -> MANUELL.OFF
    MANUELL.ON -> MANUELL.OFF : [after(30,sec) || Scheibenheizung==0]
    MANUELL.OFF -> MANUELL.ON : [Scheibenheizung==1]
  state AUTO
    state ON
      entry:SH_LED=true
    state OFF
      entry:SH_LED=false
    (default) -> AUTO.OFF
    AUTO.ON -> AUTO.OFF : [after(30,sec) || Temperatur>=2]
    AUTO.OFF -> AUTO.ON : [Temperatur<2]
  (default) -> MANUELL
  AUTO -> MANUELL : [Scheibenheizung_Auto==0]
  MANUELL -> AUTO : [Scheibenheizung_Auto==1]
  data: Scheibenheizung input; Scheibenheizung_Auto input; Temperatur input; SH_LED output
